simulink model "City_Environment_8_Cars_CS2021"  (Simulink 8.8)
settings: Solver=ode45  StartTime=0  StopTime=30  RelTol=1e-3  EnableMultiTasking=on
libraries: Solver_SF x2
settings Model: Creator=dhall  LastModifiedBy=mkhan  ExtModeTrigMode=oneshot  ExtModeArmWhenConnect=off
settings DataIOCC: LimitDataPoints=off  SignalLoggingName=sigsOut
settings OptimizationCC: BooleanDataType=off  LocalBlockOutputs=off  InitFltsAndDblsToZero=on
settings DebuggingCC: SaveWithParameterizedLinksMsg=none  SignalResolutionControl=TryResolveAllWithWarning  MultiTaskDSMMsg=warning  MultiTaskCondExecSysMsg=none  SFExecutionAtInitializationDiag=warning
settings HardwareCC: TargetBitPerPointer=64  TargetBitPerSizeT=64  TargetBitPerPtrDiffT=64  TargetLongLongMode=on  TargetIntDivRoundTo=Zero  TargetEndianess=LittleEndian  TargetWordSize=64  TargetHWDeviceType=MATLAB Host  ProdEqTarget=off
settings GRTTargetCC: TargetFcnLib=ansi_tfl_tmw.mat  CompOptLevelCompliant=off
settings ConfigComp: CovSFcnEnable=off

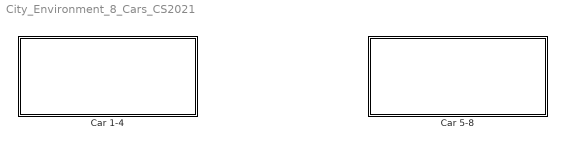
== system City_Environment_8_Cars_CS2021 ==
  Car 1-4 : Subsystem
  Car 5-8 : Subsystem

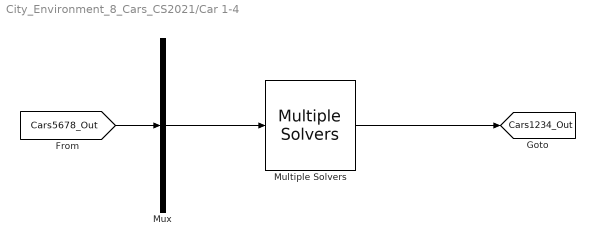
== system City_Environment_8_Cars_CS2021/Car 1-4 ==
  Multiple Solvers : Solver_SF/Multiple Solvers  Priority=1  iVehicle=1  SIMFILE=D:\product_dev\trunk\Image\CarSim\Core\CarSim_Data\Extensions\Simulink\Parallel_Solver\simfile1.sim  Run_RTs=off  vs_state_ind=Run  StopMode_ind=Vehicle Model  vs_scx=on
  Mux : Mux  Inputs=1
  tag scope: Cars1234_Out=global
  wires:
  Multiple Solvers/1 -> [Cars1234_Out]
  Mux/1 -> Multiple Solvers/1
  [Cars5678_Out] -> Mux/1

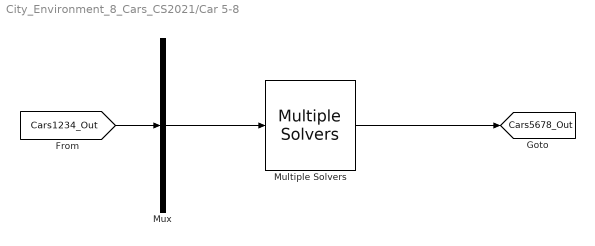
== system City_Environment_8_Cars_CS2021/Car 5-8 ==
  Multiple Solvers : Solver_SF/Multiple Solvers  Priority=1  iVehicle=2  SIMFILE=D:\product_dev\trunk\Image\CarSim\Core\CarSim_Data\Extensions\Simulink\Parallel_Solver\simfile2.sim  Run_RTs=off  vs_state_ind=Run  StopMode_ind=Vehicle Model  vs_scx=on
  Mux : Mux  Inputs=1
  tag scope: Cars5678_Out=global
  wires:
  Multiple Solvers/1 -> [Cars5678_Out]
  Mux/1 -> Multiple Solvers/1
  [Cars1234_Out] -> Mux/1
